simulink model "Ex1"  (R2021a)
settings: Solver=VariableStepAuto  StartTime=0.0  StopTime=0.05  RelTol=1e-3
settings Model: Creator=eduma  LastModifiedBy=eduma

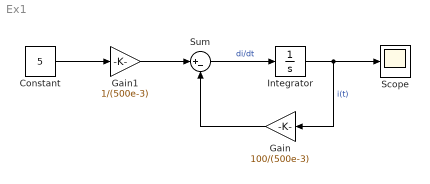
== system Ex1 ==
  Constant : Constant  Value=5
  Gain : Gain  Gain=100/(500e-3)
  Gain1 : Gain  Gain=1/(500e-3)
  Integrator : Integrator
  Scope : Scope
  Sum : Sum  Inputs=|+-
  wires:
  Sum/1 -> Integrator/1  "di/dt"
  Integrator/1 -> Scope/1, Gain/1  "i(t)"
  Gain/1 -> Sum/2
  Gain1/1 -> Sum/1
  Constant/1 -> Gain1/1
